simulink subsystem "find_id_index"  (R2021b)
settings: Solver=VariableStepAuto  StartTime=0.0  StopTime=10.0  RelTol=1e-3
values from neighbouring files (symbols this model uses):
  req_mem_size = 64    [find_id_index_testground.m]
settings Model: Creator=torha  LastModifiedBy=torha
settings SolverCC: AlgebraicLoopSolver=TrustRegion
settings DebuggingCC: SFMachineParentedDataDiag=warning

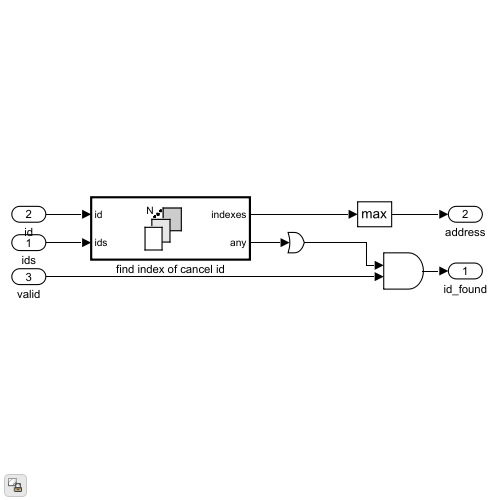
[thumbnail: Simulink's stored preview of the top-level diagram]
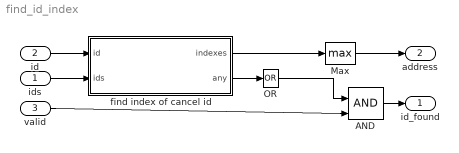
== system find_id_index ==
  ids : Inport
  id : Inport  Port=2
  valid : Inport  Port=3
  AND : Logic  IconShape=distinctive  AllPortsSameDT=off  OutDataTypeStr=boolean
  Max : MinMax  Function=max
  OR : Logic  Operator=OR  Inputs=1  IconShape=distinctive  AllPortsSameDT=off  OutDataTypeStr=boolean
  find index of cancel id : Subsystem  TreatAsAtomicUnit=on  mask{iter=fi(0:req_mem_size-1,0,log2(req_mem_size),0)}
  id_found : Outport
  address : Outport  Port=2
  wires:
  OR/1 -> AND/1
  valid/1 -> AND/2
  Max/1 -> address/1
  id/1 -> find index of cancel id/1(id)
  ids/1 -> find index of cancel id/2(ids)
  AND/1 -> id_found/1
  find index of cancel id/2(any) -> OR/1
  find index of cancel id/1(indexes) -> Max/1

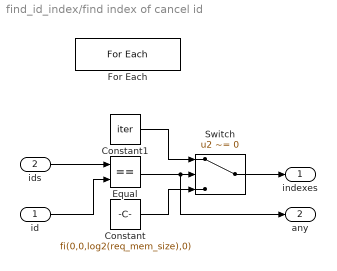
== system find_id_index/find index of cancel id ==
  id : Inport
  ids : Inport  Port=2  Partition=on  PartitionDimension=2  PartitionWidth=1  PartitionOffset=0
  Constant : Constant  Value=fi(0,0,log2(req_mem_size),0)
  Constant1 : Constant  Value=iter
  Equal : RelationalOperator  Operator===  OutDataTypeStr=boolean  RndMeth=Simplest
  For Each : ForEach  DisableCoverage=on  IterateSubsysMaskParameter=on  SubsysMaskParameterIterationDimension=2
  Switch : Switch  Criteria=u2 ~= 0
  indexes : Outport  ConcatenationDimension=1
  any : Outport  Port=2  ConcatenationDimension=1
  wires:
  Constant1/1 -> Switch/1
  ids/1 -> Equal/1
  id/1 -> Equal/2
  Equal/1 -> any/1, Switch/2
  Constant/1 -> Switch/3
  Switch/1 -> indexes/1
